simulink model "VSPSC_1"  (R2019b)
settings: Solver=ode4  StartTime=0.0  StopTime=20  FixedStep=0.0001  MaxStep=0.1  MinStep=0.001  RelTol=1e-6  AbsTol=1e-6
libraries: simulink x2
settings Model: Creator=meetn  LastModifiedBy=manth
settings SolverCC: ZeroCrossAlgorithm=Adaptive  AlgebraicLoopSolver=LineSearch
settings DebuggingCC: UnderSpecifiedDimensionMsg=warning
settings RTWCC: Description=Create Visual C/C++ Solution File for Simulink Coder  GenCodeOnly=on  TemplateMakefile=RTW.MSVCBuild  GenerateReport=on

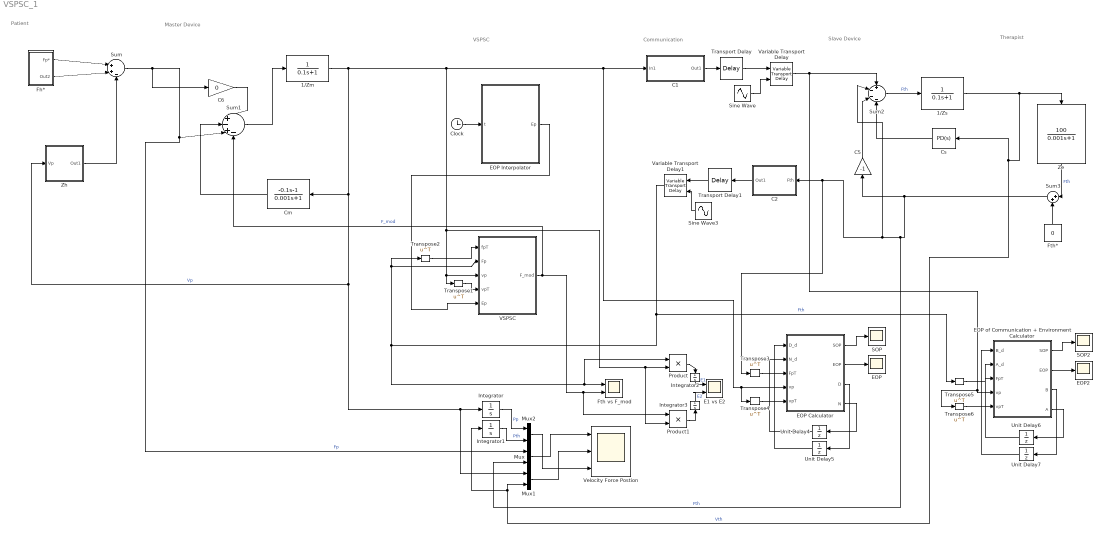
== system VSPSC_1 ==
  note: VSPSC
  note: Communication
  note: Slave Device
  note: Therapist
  note: Master Device
  note: Patient
  1/Zm : TransferFcn  Denominator=[0.1 1]
  1/Zs : TransferFcn  Denominator=[0.1 1]
  C1 : Subsystem
  C2 : Subsystem
  "C5 " : Gain  Gain=-1
  "C6 " : Gain  Gain=0
  Clock : Clock
  Cm : TransferFcn  Numerator=[-0.1 -1]  Denominator=[0.001 1]
  Cs : simulink/Continuous/PID Controller  Controller=PD  Form=Parallel  TimeDomain=Continuous-time  SampleTime=-1  IntegratorMethod=Forward Euler  FilterMethod=Forward Euler  ControllerParametersSource=internal  P=1000  I=1  D=1  UseFilter=on  N=1000  TunerSelectOption=Transfer Function Based (PID Tuner App)  InitialConditionSource=internal  InitialConditionForIntegrator=0  InitialConditionForFilter=0  DifferentiatorICPrevScaledInput=0  ExternalReset=none  TrackingMode=off  Kt=1  LimitOutput=off  UpperSaturationLimit=inf  LowerSaturationLimit=-inf  LinearizeAsGain=on  AntiWindupMode=none  Kb=1  POutMin=[]  POutMax=[]  IOutMin=[]  IOutMax=[]  DOutMin=[]  DOutMax=[]  NOutMin=[]  NOutMax=[]  SumOutMin=[]  SumOutMax=[]  SaturationOutMin=[]  SaturationOutMax=[]  PParamMin=[]  PParamMax=[]  IParamMin=[]  IParamMax=[]  DParamMin=[]  DParamMax=[]  NParamMin=[]  NParamMax=[]  KbParamMin=[]  KbParamMax=[]  KtParamMin=[]  KtParamMax=[]  KbOutMin=[]  KbOutMax=[]  KtOutMin=[]  KtOutMax=[]  IntegratorOutMin=[]  IntegratorOutMax=[]  FilterOutMin=[]  FilterOutMax=[]  SumI1OutMin=[]  SumI1OutMax=[]  SumI2OutMin=[]  SumI2OutMax=[]  SumI3OutMin=[]  SumI3OutMax=[]  SumI4OutMin=[]  SumI4OutMax=[]  SumDOutMin=[]  SumDOutMax=[]  DifferentiatorOutMin=[]  DifferentiatorOutMax=[]  FilterDiffOutCoefMin=[]  FilterDiffOutCoefMax=[]  ReciprocalOutMin=[]  ReciprocalOutMax=[]  SumDenOutMin=[]  SumDenOutMax=[]  SumNumOutMin=[]  SumNumOutMax=[]  DivideOutMin=[]  DivideOutMax=[]  IntegratorContinuousStateAttributes=''  IntegratorStateMustResolveToSignalObject=off  IntegratorRTWStateStorageClass=Auto  FilterContinuousStateAttributes=''  FilterStateMustResolveToSignalObject=off  FilterRTWStateStorageClass=Auto  ParallelPVariant=InternalParameters  IdealPVariant=Disabled  IVariant=Disabled  DVariant=InternalParameters  IntegratorVariant=Disabled  SatVariant=Disabled  AWVariant=Disabled  PCopyVariant=Disabled  TRVariant=Disabled  FdbkBlocksVariant=Forward  IdealPFdbkVariant=Disabled  SatFdbkVariant=Disabled  DerivativeFilterVariant=ContFilter  NVariant=InternalParameters  NCopyVariant=Disabled  FilterICVariant=InternalICsFilter  IntegratorICVariant=Disabled  ExternalResetVariant=Disabled  TRSumVariant=Passthrough  SumFdbkVariant=Disabled  SumVariant=Sum_PD
  E1 vs E2 : Scope  NumInputPorts=2
  EOP : Scope
  EOP Calculator : MATLAB Function  TreatAsAtomicUnit=on
  EOP Interpolator : MATLAB Function  TreatAsAtomicUnit=on
  EOP of Communication + Environment Calculator : MATLAB Function  TreatAsAtomicUnit=on
  EOP2 : Scope
  Fh* : Subsystem
  Fth vs F_mod : Scope  NumInputPorts=2
  Fth* : Constant  Value=0  OutDataTypeStr=Inherit: Inherit via back propagation
  Integrator{,1..3} (4 alike) : Integrator
  Mux : Mux  Inputs=2
  Mux1 : Mux  Inputs=2
  Mux2 : Mux  Inputs=2
  Product : Product
  Product1 : Product
  SOP : Scope
  SOP2 : Scope
  Sine Wave : Sin  Amplitude=0.02  Frequency=12  SampleTime=0
  Sine Wave3 : Sin  Amplitude=0.02  Frequency=12  SampleTime=0
  Sum : Sum  Inputs=|++-
  Sum1 : Sum  Inputs=|+-+-
  Sum2 : Sum  Inputs=+---
  Sum3 : Sum  Inputs=|++
  Transport Delay : TransportDelay  DelayTime=0.1  PadeOrder=3
  Transport Delay1 : TransportDelay  DelayTime=0.1  PadeOrder=3
  Transpose{1..6} (6 alike) : Math  Operator=transpose  SignedPower=off  SaturateOnIntegerOverflow=on
  Unit Delay{4..7} (4 alike) : UnitDelay  SampleTime=-1  HasFrameUpgradeWarning=on
  VSPSC : MATLAB Function  TreatAsAtomicUnit=on
  Variable Transport Delay : VariableTransportDelay  PadeOrder=3
  Variable Transport Delay1 : VariableTransportDelay  PadeOrder=3
  Velocity Force Postion : Scope  NumInputPorts=3
  Ze : TransferFcn  Numerator=[100]  Denominator=[0.001 1]
  Zh : Subsystem
  wires:
  "C6 "/1 -> Sum1/1
  Cs/1 -> Sum2/4
  Ze/1 -> Sum3/1  "Fth"
  Sum1/1 -> 1/Zm/1
  Fth*/1 -> Sum3/2
  1/Zs/1 -> Ze/1, Cs/1, Integrator1/1, Mux1/2  "Vth"
  Sum2/1 -> 1/Zs/1  "Fth"
  Sum/1 -> "C6 "/1, Mux/1, Sum1/3  "Fp"
  "C5 "/1 -> Sum2/3
  Cm/1 -> Sum1/2
  Sum3/1 -> Transpose3/1, C2/1(Fth), Sum2/2, Mux/2, "C5 "/1  "Fth"
  Mux/1 -> Velocity Force Postion/1
  Mux1/1 -> Velocity Force Postion/2
  VSPSC/1(F_mod) -> Sum1/4, Product1/1, Fth vs F_mod/2  "F_mod"
  Variable Transport Delay1/1 -> Transpose2/1, VSPSC/2(Fp), Product/1, Fth vs F_mod/1, Transpose5/1  "Fth"
  Mux2/1 -> Velocity Force Postion/3
  Integrator/1 -> Mux2/1  "Pp"
  Integrator1/1 -> Mux2/2  "Pth"
  Sine Wave/1 -> Variable Transport Delay/2
  Transport Delay/1 -> Variable Transport Delay/1
  C1/1(Out1) -> Transport Delay/1
  Sine Wave3/1 -> Variable Transport Delay1/2
  Transport Delay1/1 -> Variable Transport Delay1/1
  C2/1(Out1) -> Transport Delay1/1
  Fh*/1(Fp*) -> Sum/1
  Fh*/2(Out2) -> Sum/2
  Zh/1(Out1) -> Sum/3
  Transpose1/1 -> VSPSC/4(vpT)
  Transpose2/1 -> VSPSC/1(fpT)
  Product/1 -> Integrator2/1
  Product1/1 -> Integrator3/1
  Integrator2/1 -> E1 vs E2/1  "E1"
  Integrator3/1 -> E1 vs E2/2  "E2"
  Clock/1 -> EOP Interpolator/1(t)
  EOP Interpolator/1(Ep) -> VSPSC/5(Ep)
  EOP Calculator/3(D) -> Unit Delay5/1
  Transpose4/1 -> EOP Calculator/5(vpT)
  1/Zm/1 -> Mux1/1, Integrator/1, Zh/1(Vp), Cm/1, VSPSC/3(vp), Transpose1/1, Product1/2, Product/2, EOP Calculator/4(vp), Transpose4/1, C1/1(In1)  "Vp"
  Transpose3/1 -> EOP Calculator/3(FpT)
  Unit Delay5/1 -> EOP Calculator/1(D_d)
  EOP Calculator/1(SOP) -> SOP/1
  EOP Calculator/2(EOP) -> EOP/1
  EOP Calculator/4(N) -> Unit Delay4/1
  Unit Delay4/1 -> EOP Calculator/2(N_d)
  EOP of Communication + Environment Calculator/1(SOP) -> SOP2/1
  Transpose6/1 -> EOP of Communication + Environment Calculator/5(vpT)
  Unit Delay6/1 -> EOP of Communication + Environment Calculator/2(A_d)
  Unit Delay7/1 -> EOP of Communication + Environment Calculator/1(B_d)
  Variable Transport Delay/1 -> Transpose6/1, EOP of Communication + Environment Calculator/4(vp), Sum2/1
  EOP of Communication + Environment Calculator/2(EOP) -> EOP2/1
  Transpose5/1 -> EOP of Communication + Environment Calculator/3(FpT)
  EOP of Communication + Environment Calculator/3(B) -> Unit Delay7/1
  EOP of Communication + Environment Calculator/4(A) -> Unit Delay6/1

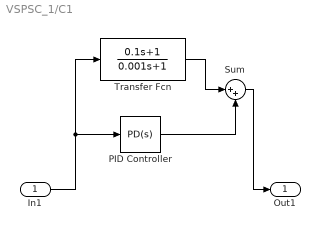
== system VSPSC_1/C1 ==
  In1 : Inport
  PID Controller : simulink/Continuous/PID Controller  Controller=PD  Form=Parallel  TimeDomain=Continuous-time  SampleTime=-1  IntegratorMethod=Forward Euler  FilterMethod=Forward Euler  ControllerParametersSource=internal  P=1000  I=1  D=1  UseFilter=on  N=1000  TunerSelectOption=Transfer Function Based (PID Tuner App)  InitialConditionSource=internal  InitialConditionForIntegrator=0  InitialConditionForFilter=0  DifferentiatorICPrevScaledInput=0  ExternalReset=none  TrackingMode=off  Kt=1  LimitOutput=off  UpperSaturationLimit=inf  LowerSaturationLimit=-inf  LinearizeAsGain=on  AntiWindupMode=none  Kb=1  POutMin=[]  POutMax=[]  IOutMin=[]  IOutMax=[]  DOutMin=[]  DOutMax=[]  NOutMin=[]  NOutMax=[]  SumOutMin=[]  SumOutMax=[]  SaturationOutMin=[]  SaturationOutMax=[]  PParamMin=[]  PParamMax=[]  IParamMin=[]  IParamMax=[]  DParamMin=[]  DParamMax=[]  NParamMin=[]  NParamMax=[]  KbParamMin=[]  KbParamMax=[]  KtParamMin=[]  KtParamMax=[]  KbOutMin=[]  KbOutMax=[]  KtOutMin=[]  KtOutMax=[]  IntegratorOutMin=[]  IntegratorOutMax=[]  FilterOutMin=[]  FilterOutMax=[]  SumI1OutMin=[]  SumI1OutMax=[]  SumI2OutMin=[]  SumI2OutMax=[]  SumI3OutMin=[]  SumI3OutMax=[]  SumI4OutMin=[]  SumI4OutMax=[]  SumDOutMin=[]  SumDOutMax=[]  DifferentiatorOutMin=[]  DifferentiatorOutMax=[]  FilterDiffOutCoefMin=[]  FilterDiffOutCoefMax=[]  ReciprocalOutMin=[]  ReciprocalOutMax=[]  SumDenOutMin=[]  SumDenOutMax=[]  SumNumOutMin=[]  SumNumOutMax=[]  DivideOutMin=[]  DivideOutMax=[]  IntegratorContinuousStateAttributes=''  IntegratorStateMustResolveToSignalObject=off  IntegratorRTWStateStorageClass=Auto  FilterContinuousStateAttributes=''  FilterStateMustResolveToSignalObject=off  FilterRTWStateStorageClass=Auto  ParallelPVariant=InternalParameters  IdealPVariant=Disabled  IVariant=Disabled  DVariant=InternalParameters  IntegratorVariant=Disabled  SatVariant=Disabled  AWVariant=Disabled  PCopyVariant=Disabled  TRVariant=Disabled  FdbkBlocksVariant=Forward  IdealPFdbkVariant=Disabled  SatFdbkVariant=Disabled  DerivativeFilterVariant=ContFilter  NVariant=InternalParameters  NCopyVariant=Disabled  FilterICVariant=InternalICsFilter  IntegratorICVariant=Disabled  ExternalResetVariant=Disabled  TRSumVariant=Passthrough  SumFdbkVariant=Disabled  SumVariant=Sum_PD
  Sum : Sum  Inputs=|++
  Transfer Fcn : TransferFcn  Numerator=[0.1 1]  Denominator=[0.001 1]
  Out1 : Outport
  wires:
  In1/1 -> PID Controller/1, Transfer Fcn/1
  Transfer Fcn/1 -> Sum/1
  PID Controller/1 -> Sum/2
  Sum/1 -> Out1/1

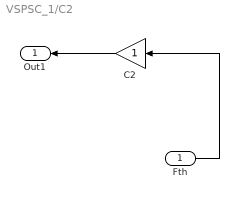
== system VSPSC_1/C2 ==
  Fth : Inport
  C2 : Gain
  Out1 : Outport
  wires:
  Fth/1 -> C2/1
  C2/1 -> Out1/1

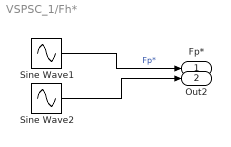
== system VSPSC_1/Fh* ==
  Sine Wave1 : Sin  Frequency=5  SampleTime=0
  Sine Wave2 : Sin  Frequency=8  Phase=pi/2  SampleTime=0
  Fp* : Outport
  Out2 : Outport  Port=2
  wires:
  Sine Wave1/1 -> Fp*/1  "Fp*"
  Sine Wave2/1 -> Out2/1

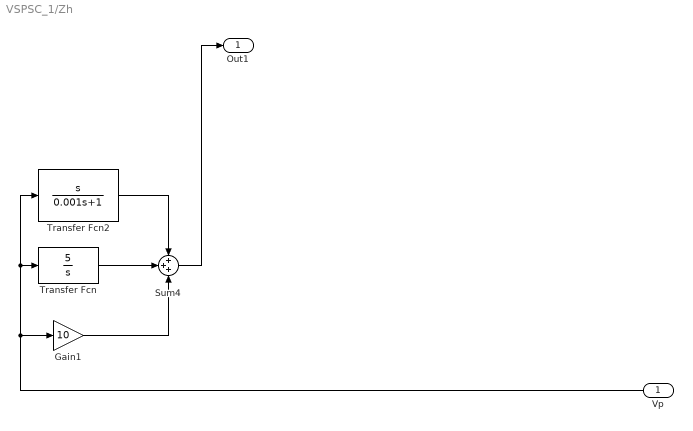
== system VSPSC_1/Zh ==
  Vp : Inport
  Gain1 : Gain  Gain=10
  Sum4 : Sum  Inputs=3
  Transfer Fcn : TransferFcn  Numerator=[5]  Denominator=[1 0]
  Transfer Fcn2 : TransferFcn  Numerator=[1 0]  Denominator=[0.001 1]
  Out1 : Outport
  wires:
  Vp/1 -> Gain1/1, Transfer Fcn/1, Transfer Fcn2/1
  Sum4/1 -> Out1/1
  Transfer Fcn/1 -> Sum4/2
  Transfer Fcn2/1 -> Sum4/1
  Gain1/1 -> Sum4/3

== matlab function VSPSC_1/EOP Interpolator ==
  data: t input; Ep output
function Ep  = Stabilizer(t)


if t<=10
Ep = 3;
else
    Ep=6;
end

== matlab function VSPSC_1/VSPSC ==
  data: fpT input; Fp input; F_mod output; vp input; vpT input; Ep input
function F_mod  = Stabilizer(fpT,Fp,vp,vpT,Ep)


if abs(Ep*vpT*vp)>=abs(fpT*vp)
s=Fp;
else
    s=((abs(Ep*vp))*Fp)/(abs(Fp)+0.00001)+0.00001;
end


if (fpT*vp)>=0
FRG=Fp;
else
    FRG=s;
end

F_mod= 1*FRG+0.00001;

== matlab function VSPSC_1/EOP Calculator ==
  data: D_d input; N_d input; SOP output; EOP output; FpT input; vp input; vpT input; D output; N output
function [SOP,EOP,D,N] = EOP_Calculator(D_d,N_d,FpT,vp,vpT)

N=N_d+0.001*(FpT*vp);
D=D_d+0.001*(vpT*vp);
 
SOP=N/D;
 
EOP=-SOP;

== matlab function VSPSC_1/EOP of Communication + Environment Calculator ==
  data: B_d input; A_d input; SOP output; EOP output; FpT input; vp input; vpT input; B output; A output
function [SOP,EOP,B,A] = EOP_Calculator(B_d,A_d,FpT,vp,vpT)

A=A_d+0.001*(FpT*vp);
B=B_d+0.001*(vpT*vp);
 
SOP=A/B;
 
EOP=-SOP;
